simulink model "observer_test"  (R2019a)
settings: Solver=VariableStepAuto  StartTime=0.0  StopTime=11  RelTol=1e-3
settings Model: Creator=harkib  LastModifiedBy=harki
settings DataIOCC: ReturnWorkspaceOutputs=off
settings DebuggingCC: PregeneratedLibrarySubsystemCodeDiagnostic=none  ArithmeticOperatorsInVariantConditions=warning
settings SFSimCC: SimUseLocalCustomCode=off
settings RTWCC: RTWUseLocalCustomCode=off

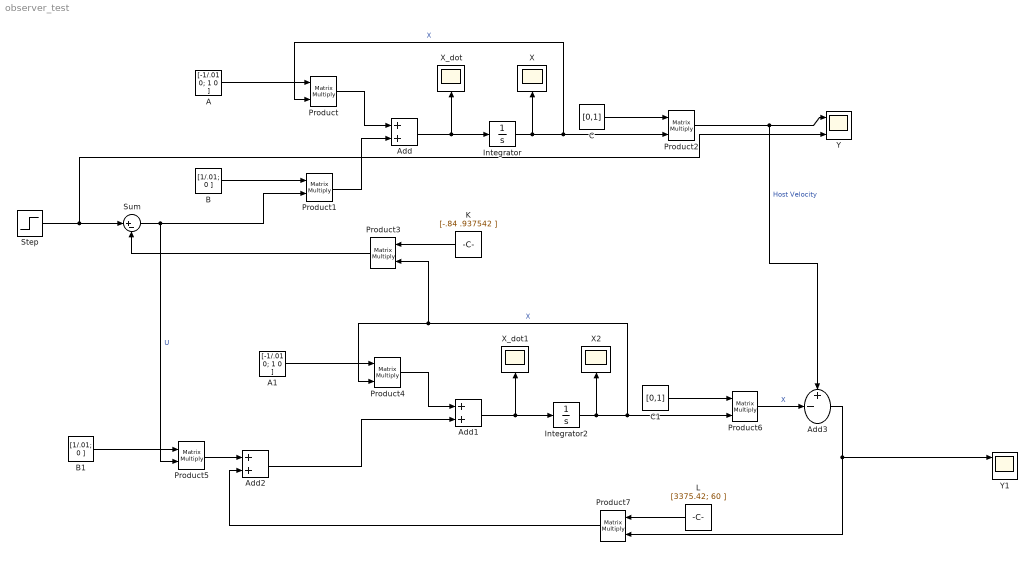
== system observer_test ==
  A : Constant  Value=[-1/.01 0; 1 0 ]  VectorParams1D=off
  A1 : Constant  Value=[-1/.01 0; 1 0 ]  VectorParams1D=off
  Add : Sum
  Add1 : Sum
  Add2 : Sum
  Add3 : Sum  Inputs=+-|
  B : Constant  Value=[1/.01; 0 ]  VectorParams1D=off
  B1 : Constant  Value=[1/.01; 0 ]  VectorParams1D=off
  C : Constant  Value=[0,1]  VectorParams1D=off
  C1 : Constant  Value=[0,1]  VectorParams1D=off
  Integrator : Integrator
  Integrator2 : Integrator
  K : Constant  Value=[-.84 .937542 ]  VectorParams1D=off
  L : Constant  Value=[3375.42; 60 ]  VectorParams1D=off
  Product{,1..7} (8 alike) : Product  Multiplication=Matrix(*)
  Step : Step  SampleTime=0
  Sum : Sum  Inputs=|+-
  X : Scope
  X2 : Scope
  X_dot : Scope
  X_dot1 : Scope
  Y : Scope  NumInputPorts=3
  Y1 : Scope  NumInputPorts=3
  wires:
  Add/1 -> X_dot/1, Integrator/1
  Product1/1 -> Add/2
  Product/1 -> Add/1
  B/1 -> Product1/1
  A/1 -> Product/1
  K/1 -> Product3/1
  Integrator/1 -> Product2/2, Product/2, X/1  "X"
  Product3/1 -> Sum/2
  Sum/1 -> Product5/2, Product1/2  "U"
  C/1 -> Product2/1
  Product2/1 -> Add3/1, Y/1  "Host Velocity"
  Add1/1 -> X_dot1/1, Integrator2/1
  Product4/1 -> Add1/1
  Integrator2/1 -> Product6/2, Product3/2, Product4/2, X2/1  "X"
  C1/1 -> Product6/1
  A1/1 -> Product4/1
  Add2/1 -> Add1/2
  B1/1 -> Product5/1
  Product5/1 -> Add2/1
  L/1 -> Product7/1
  Product7/1 -> Add2/2
  Product6/1 -> Add3/2  "X"
  Add3/1 -> Product7/2, Y1/1
  Step/1 -> Y/3, Sum/1
